simulink model "clase19012021_1"  (R2020b)
settings: Solver=VariableStepAuto  StartTime=0.0  StopTime=50/100  RelTol=1e-3
libraries: commdigbbndfm2 x1, commrandsrc3 x1
settings Model: Creator=fernando  LastModifiedBy=fernando

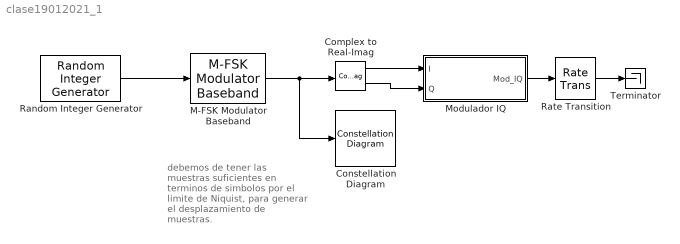
== system clase19012021_1 ==
  note: debemos de tener las muestras suficientes en terminos de simbolos por el limite de Niquist, para generar el desplazamiento de muestras.
  Complex to Real-Imag : ComplexToRealImag
  Constellation Diagram : ConstellationDiagram
  M-FSK Modulator Baseband : commdigbbndfm2/M-FSK Modulator Baseband  M=2  InType=Bit  Enc=Gray  freqSep=1e3  phaseType=Continuous  numSamp=100  RateOptions=Enforce single-rate processing  outDataType=double
  Modulador IQ : Subsystem
  Random Integer Generator : commrandsrc3/Random Integer Generator  SetSize=2  SeedSource=Auto  Seed=0  SampleTime=1/500  SamplesPerFrame=1  OutputDataType=boolean  SimulateUsing=Interpreted execution
  Rate Transition : RateTransition  OutPortSampleTime=1/8e3/10
  Terminator : Terminator
  wires:
  Modulador IQ/1(Mod_IQ) -> Rate Transition/1
  Complex to Real-Imag/2 -> Modulador IQ/2(Q)
  Complex to Real-Imag/1 -> Modulador IQ/1(I)
  M-FSK Modulator Baseband/1 -> Constellation Diagram/1, Complex to Real-Imag/1
  Rate Transition/1 -> Terminator/1
  Random Integer Generator/1 -> M-FSK Modulator Baseband/1

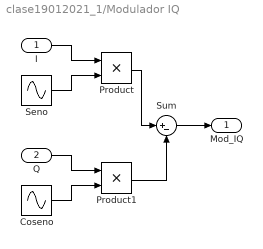
== system clase19012021_1/Modulador IQ ==
  I : Inport
  Q : Inport  Port=2
  Coseno : Sin  Frequency=2*pi*1e3  Phase=pi/2  SampleTime=0
  Product : Product
  Product1 : Product
  Seno : Sin  Frequency=2*pi*1e3  SampleTime=0
  Sum : Sum  Inputs=|+-
  Mod_IQ : Outport
  wires:
  Seno/1 -> Product/2
  I/1 -> Product/1
  Coseno/1 -> Product1/2
  Product1/1 -> Sum/2
  Sum/1 -> Mod_IQ/1
  Product/1 -> Sum/1
  Q/1 -> Product1/1
